simulink model "Ball_and_Plate_MicroLabBox_student"  (R2019b)
settings: Solver=ode1  StartTime=0.0  StopTime=Inf  FixedStep=0.001  RelTol=1e-3
PostLoadFcn:
  | , if any(exist('dsrtsu_mdlpostloadfcn', 'file') ~= 0), dsrtsu_mdlpostloadfcn('Execute', bdroot); end,
InitFcn:
  | , if any(exist('rtifpga_mdlclblib', 'file') ~= 0), rtifpga_mdlclblib('Init', bdroot); end,
undefined symbols (not defined in the file): A_obs, A_robust, B_obs, B_robust, ball_pos_sat, ball_vel_sat, C_obs, C_robust, D_obs, D_robust, g, K_lqr, path, plate_angle_sat, Q_kf, R_kf, Ts_fast, Ts_Inner, Ts_Outer, uA, uB, uC
libraries: rtiemclib x6, simulink x3, rtiethernetlib x3, rti1202lib_dac_class1 x3, mpclib x1
(part 3 of 3)

== matlab function Ball_and_Plate_MicroLabBox_student/Innerloop_Actuator/Motor_A/MATLAB Function ==
  data: e input; u output; reset_integrator input
function u = fcn(e, reset_integrator)
% You need to fill here

u = 0;

== matlab function Ball_and_Plate_MicroLabBox_student/Innerloop_Actuator/Motor_C/MATLAB Function ==
  data: e input; u output; reset_integrator input
function u = fcn(e, reset_integrator)
% You need to fill here

u = 0;

== matlab function Ball_and_Plate_MicroLabBox_student/Innerloop_Actuator/Motor_B/MATLAB Function1 ==
  data: e input; u output; reset_integrator input
function u = fcn(e, reset_integrator)
% You need to fill here

u = 0;

== matlab function Ball_and_Plate_MicroLabBox_student/Innerloop_Actuator/Motor_A/Multisine/MATLAB Function ==
  data: enable input; u input; y output
function y = Multisine_id(enable, u)

persistent index previous_enable

% Initialize
if isempty(index)
    index = 1;
end

if isempty(previous_enable)
    previous_enable = 0;
end

N = length(u);

% Detect rising edge (re-enable)
if enable && ~previous_enable
    index = 1;
end

% Output logic
if enable

    % If still inside signal → output sample
    if index <= N
        y = u(index);
        index = index + 1;

    else
        % Signal finished → output zero
        y = 0;
    end

else
    % Disabled → output zero
    y = 0;
end

previous_enable = enable;

== matlab function Ball_and_Plate_MicroLabBox_student/Innerloop_Actuator/Motor_B/Multisine/MATLAB Function ==
  data: enable input; u input; y output
function y = Multisine_id(enable, u)

persistent index previous_enable

% Initialize
if isempty(index)
    index = 1;
end

if isempty(previous_enable)
    previous_enable = 0;
end

N = length(u);

% Detect rising edge (re-enable)
if enable && ~previous_enable
    index = 1;
end

% Output logic
if enable

    % If still inside signal → output sample
    if index <= N
        y = u(index);
        index = index + 1;

    else
        % Signal finished → output zero
        y = 0;
    end

else
    % Disabled → output zero
    y = 0;
end

previous_enable = enable;

== matlab function Ball_and_Plate_MicroLabBox_student/Innerloop_Actuator/Motor_C/Multisine/MATLAB Function ==
  data: enable input; u input; y output
function y = Multisine_id(enable, u)

persistent index previous_enable

% Initialize
if isempty(index)
    index = 1;
end

if isempty(previous_enable)
    previous_enable = 0;
end

N = length(u);

% Detect rising edge (re-enable)
if enable && ~previous_enable
    index = 1;
end

% Output logic
if enable

    % If still inside signal → output sample
    if index <= N
        y = u(index);
        index = index + 1;

    else
        % Signal finished → output zero
        y = 0;
    end

else
    % Disabled → output zero
    y = 0;
end

previous_enable = enable;

== matlab function Ball_and_Plate_MicroLabBox_student/coordinates_ball ==
  data: x_2_pixels input; x_2 output; y_2_pixels input; y_2 output; theta_1 input; theta_2 input
function [x_2, y_2] = fcn(x_2_pixels, y_2_pixels, theta_1, theta_2)
    %A01_fun
    %    OUT1 = A01_fun(THETA_1,THETA_2)
    
    %    This function was generated by the Symbolic Math Toolbox version 9.3.
    %    22-May-2025 12:09:11
    y_offset = 242.82;
    x_offset = 295.83;
    conversion_factor = 1120.25;
%     ball_radius = 20e-3;%mm
    x_2_e0 = (double(x_2_pixels)-x_offset)/conversion_factor;
    y_2_e0 = (double(y_2_pixels)-y_offset)/conversion_factor;
    t2 = cos(theta_1);
    t3 = cos(theta_2);
    t4 = sin(theta_1);
    t5 = sin(theta_2);
    out1 = reshape([t3,t4.*t5,-t2.*t5,0.0,t2,t4,t5,-t3.*t4,t2.*t3],[3,3]);
%     temp = double([x_2_e0, y_2_e0, -ball_radius])*double(out1);
    x_2 = x_2_e0;%temp(1);
    y_2 = y_2_e0;%temp(2);
end

== matlab function Ball_and_Plate_MicroLabBox_student/Innerloop_Actuator/Motor_C/Multisine1/MATLAB Function ==
  data: enable input; u input; y output
function y = Multisine_id(enable, u)

persistent index previous_enable

% Initialize
if isempty(index)
    index = 1;
end

if isempty(previous_enable)
    previous_enable = 0;
end

N = length(u);

% Detect rising edge (re-enable)
if enable && ~previous_enable
    index = 1;
end

% Output logic
if enable

    % If still inside signal → output sample
    if index <= N
        y = u(index);
        index = index + 1;

    else
        % Signal finished → output zero
        y = 0;
    end

else
    % Disabled → output zero
    y = 0;
end

previous_enable = enable;

== matlab function Ball_and_Plate_MicroLabBox_student/Innerloop_Actuator/Motor_B/Init_motion/MATLAB Function1 ==
  data: reference_end input; path output; end_time input; Ts input; measured_position input
function path = Quintic_Polynomial_Trajectory_Time(reference_end, end_time, Ts, measured_position)
%% Quintic_Polynomial_Trajectory(reference_end, average_velocity)
% This function outputs a quintic polynomial trajectory over time in 
% Simulink given the end reference and average velocity. The starting 
% velocity and acceleration are set to zero.
%
% Input Arguments
% reference_end = desired end position of the trajectory
% end_time = end time of trajectory; for every new input 
% trajectory starts at time 0 and ends at end_time
% measured_position = current position of the robot arm
%
% Output Arguments
% path = path of the trajectory over time
%
% Quinten Swaan 17-08-2022
%
% Control Systems Technology group
% Departement of Mechanical Engineering
% Eindhoven University of Technology


persistent previous_value_reference_start previous_value_reference_end ...
    path_array index 

if isempty(previous_value_reference_start)
    previous_value_reference_start = 0;
end

if isempty(previous_value_reference_end)
    previous_value_reference_end = 0;
end

if isempty(path_array)
    path_array = zeros(1,1);
end

if isempty(index)
    index = 1;
end


% Obtain new trajectory if a new end reference is given
if previous_value_reference_end ~= reference_end
    t0 = 0;                                 %Starting time
    q0 = previous_value_reference_start;    %Starting position
    v0 = 0;                                 %Starting velocity
    ac0 = 0;                                %Starting acceleration
    tf = end_time;                          %End time
    qf = reference_end;                     %End position
    vf = 0;                                 %End velocity
    acf = 0;                                %End acceleration

    M = [1 t0 t0^2 t0^3 t0^4 t0^5;
    0 1 2*t0 3*t0^2 4*t0^3 5*t0^4;
    0 0 2 6*t0 12*t0^2 20*t0^3;
    1 tf tf^2 tf^3 tf^4 tf^5;
    0 1 2*tf 3*tf^2 4*tf^3 5*tf^4;
    0 0 2 6*tf 12*tf^2 20*tf^3];

    b = [q0; v0; ac0; qf; vf; acf];

    x = M \ b;

    t = t0:Ts:tf;

    path_array = x(1) + x(2).*t + x(3).*t.^2 + x(4).*t.^3 + +x(5).*t.^4 + x(6).*t.^5;

    index = 1;
    reference_current = path_array(index);

% Output the reference per timestep
else
    if index < length(path_array)
        index = index + 1;
    end
    reference_current = path_array(index);
end

previous_value_reference_end = reference_end;
previous_value_reference_start = measured_position;

path = reference_current;

== matlab function Ball_and_Plate_MicroLabBox_student/Innerloop_Actuator/Motor_B/Init_motion/MATLAB Function2 ==
  data: y input; path output; start input; init_value input; current_pos input
function path = init_motion(y, start, init_value, current_pos)

if start > 0.5
    path = init_value;
elseif start < 0.5
    path = y;
else 
    path = 0;
end

== matlab function Ball_and_Plate_MicroLabBox_student/Innerloop_Actuator/Motor_C/Init_motion/MATLAB Function1 ==
  data: reference_end input; path output; end_time input; Ts input; measured_position input
function path = Quintic_Polynomial_Trajectory_Time(reference_end, end_time, Ts, measured_position)
%% Quintic_Polynomial_Trajectory(reference_end, average_velocity)
% This function outputs a quintic polynomial trajectory over time in 
% Simulink given the end reference and average velocity. The starting 
% velocity and acceleration are set to zero.
%
% Input Arguments
% reference_end = desired end position of the trajectory
% end_time = end time of trajectory; for every new input 
% trajectory starts at time 0 and ends at end_time
% measured_position = current position of the robot arm
%
% Output Arguments
% path = path of the trajectory over time
%
% Quinten Swaan 17-08-2022
%
% Control Systems Technology group
% Departement of Mechanical Engineering
% Eindhoven University of Technology


persistent previous_value_reference_start previous_value_reference_end ...
    path_array index 

if isempty(previous_value_reference_start)
    previous_value_reference_start = 0;
end

if isempty(previous_value_reference_end)
    previous_value_reference_end = 0;
end

if isempty(path_array)
    path_array = zeros(1,1);
end

if isempty(index)
    index = 1;
end


% Obtain new trajectory if a new end reference is given
if previous_value_reference_end ~= reference_end
    t0 = 0;                                 %Starting time
    q0 = previous_value_reference_start;    %Starting position
    v0 = 0;                                 %Starting velocity
    ac0 = 0;                                %Starting acceleration
    tf = end_time;                          %End time
    qf = reference_end;                     %End position
    vf = 0;                                 %End velocity
    acf = 0;                                %End acceleration

    M = [1 t0 t0^2 t0^3 t0^4 t0^5;
    0 1 2*t0 3*t0^2 4*t0^3 5*t0^4;
    0 0 2 6*t0 12*t0^2 20*t0^3;
    1 tf tf^2 tf^3 tf^4 tf^5;
    0 1 2*tf 3*tf^2 4*tf^3 5*tf^4;
    0 0 2 6*tf 12*tf^2 20*tf^3];

    b = [q0; v0; ac0; qf; vf; acf];

    x = M \ b;

    t = t0:Ts:tf;

    path_array = x(1) + x(2).*t + x(3).*t.^2 + x(4).*t.^3 + +x(5).*t.^4 + x(6).*t.^5;

    index = 1;
    reference_current = path_array(index);

% Output the reference per timestep
else
    if index < length(path_array)
        index = index + 1;
    end
    reference_current = path_array(index);
end

previous_value_reference_end = reference_end;
previous_value_reference_start = measured_position;

path = reference_current;

== matlab function Ball_and_Plate_MicroLabBox_student/Innerloop_Actuator/Motor_C/Init_motion/MATLAB Function2 ==
  data: y input; path output; start input; init_value input; current_pos input
function path = init_motion(y, start, init_value, current_pos)

if start > 0.5
    path = init_value;
elseif start < 0.5
    path = y;
else 
    path = 0;
end

== matlab function Ball_and_Plate_MicroLabBox_student/Innerloop_Actuator/Motor_A/Init_motion/MATLAB Function ==
  data: enable input; u input; y output
function y = init_motion(enable, u)

persistent index previous_enable

% Initialize
if isempty(index)
    index = 1;
end

if isempty(previous_enable)
    previous_enable = 0;
end

N = length(u);

% Detect rising edge (re-enable)
if enable && ~previous_enable
    index = 1;
end

% Output logic
if enable

    % If still inside signal → output sample
    if index <= N
        y = u(index);
        index = index + 1;

    else
        % Signal finished → output zero
        y = 0;
    end

else
    % Disabled → output zero
    y = -0.0289;
end

previous_enable = enable;

== matlab function Ball_and_Plate_MicroLabBox_student/Innerloop_Actuator/Motor_B/Init_motion/MATLAB Function ==
  data: enable input; u input; y output
function y = init_motion(enable, u)

persistent index previous_enable

% Initialize
if isempty(index)
    index = 1;
end

if isempty(previous_enable)
    previous_enable = 0;
end

N = length(u);

% Detect rising edge (re-enable)
if enable && ~previous_enable
    index = 1;
end

% Output logic
if enable

    % If still inside signal → output sample
    if index <= N
        y = u(index);
        index = index + 1;

    else
        % Signal finished → output zero
        y = 0;
    end

else
    % Disabled → output zero
    y = -0.0289;
end

previous_enable = enable;

== matlab function Ball_and_Plate_MicroLabBox_student/Innerloop_Actuator/Motor_C/Init_motion/MATLAB Function ==
  data: enable input; u input; y output
function y = init_motion(enable, u)

persistent index previous_enable

% Initialize
if isempty(index)
    index = 1;
end

if isempty(previous_enable)
    previous_enable = 0;
end

N = length(u);

% Detect rising edge (re-enable)
if enable && ~previous_enable
    index = 1;
end

% Output logic
if enable

    % If still inside signal → output sample
    if index <= N
        y = u(index);
        index = index + 1;

    else
        % Signal finished → output zero
        y = 0;
    end

else
    % Disabled → output zero
    y = -0.0289;
end

previous_enable = enable;

== matlab function Ball_and_Plate_MicroLabBox_student/Innerloop_Actuator/AngleToPos  ==
  data: alpha input; pos1 output; beta input; psi input; pos2 output; pos3 output
function [pos1, pos2, pos3] = angleToPos(alpha, beta, psi)
    % Returns the actuator positions required to reach the desired angle
    % note: the position is absolute in the global frame

    % Physical Constants
    r = 0.17;           % Joint radius (m)
    T = [0; 0; 0.322];  % Resting height vector (m)
    
    % Joint positions on base and plate (equilateral triangle)
    % These match the definitions in your posToAngle function
    theta = [0, deg2rad(240), deg2rad(120)];
    B = [r*cos(theta); r*sin(theta); zeros(1,3)]; % Base joints (b_i)
    P = [r*cos(theta); r*sin(theta); zeros(1,3)]; % Plate joints (p_i)
    
    % Rotation Matrices (Yaw-Pitch-Roll order)
    Rz = [cos(psi) -sin(psi) 0; sin(psi) cos(psi) 0; 0 0 1];
    Ry = [cos(beta) 0 sin(beta); 0 1 0; -sin(beta) 0 cos(beta)];
    Rx = [1 0 0; 0 cos(alpha) -sin(alpha); 0 sin(alpha) cos(alpha)];
    R_BtoP = Rz * Ry * Rx; 
    
    % Compute absolute position for each motor
    % Motor 1
    l1_vec = T + (R_BtoP * P(:,1)) - B(:,1);
    pos1 = norm(l1_vec);
    
    % Motor 2
    l2_vec = T + (R_BtoP * P(:,2)) - B(:,2);
    pos2 = norm(l2_vec);
    
    % Motor 3
    l3_vec = T + (R_BtoP * P(:,3)) - B(:,3);
    pos3 = norm(l3_vec);
end

== matlab function Ball_and_Plate_MicroLabBox_student/Innerloop_Actuator/Motor_A/MATLAB Function1 ==
  data: reference_end input; path output; end_time input; Ts input; measured_position input
function path = Quintic_Time(reference_end, end_time, Ts, measured_position)
% QUINTIC_POLYNOMIAL_TRAJECTORY_TIME
% Calculated analytically per step to be compatible with dSPACE/Control Desk.

% Persistent variables to store coefficients and the "internal clock"
persistent coeffs t_elapsed prev_ref_end tf_internal
if isempty(coeffs)
    coeffs = zeros(6, 1); % a0, a1, a2, a3, a4, a5
end
if isempty(t_elapsed)
    t_elapsed = 0;
end
if isempty(prev_ref_end)
    prev_ref_end = reference_end;
end
if isempty(tf_internal)
    tf_internal = 0;
end

% Check if a new trajectory is requested
if reference_end ~= prev_ref_end
    % Reset timer
    t_elapsed = 0;
    tf_internal = end_time;
    
    % Boundary conditions
    q0 = prev_ref_end; 
    qf = reference_end;
    v0 = 0; vf = 0;
    ac0 = 0; acf = 0;
    
    % Solver for t0 = 0
    % We solve the system: M * coeffs = b
    % Using tf_internal instead of end_time to ensure consistency during the run
    T = tf_internal;
    M = [1, 0, 0,  0,    0,    0;
         0, 1, 0,  0,    0,    0;
         0, 0, 2,  0,    0,    0;
         1, T, T^2, T^3,  T^4,  T^5;
         0, 1, 2*T, 3*T^2, 4*T^3, 5*T^4;
         0, 0, 2,   6*T,   12*T^2, 20*T^3];
     
    b = [q0; v0; ac0; qf; vf; acf];
    
    % Calculate coefficients (Matrix is small 6x6, so this is fast)
    coeffs = M \ b;
end

% Calculate current reference based on elapsed time
t = t_elapsed;

if t <= tf_internal
    % Quintic Equation: path = a0 + a1*t + a2*t^2 + a3*t^3 + a4*t^4 + a5*t^5
    path = coeffs(1) + coeffs(2)*t + coeffs(3)*t^2 + coeffs(4)*t^3 + coeffs(5)*t^4 + coeffs(6)*t^5;
    
    % Increment time for the next step
    t_elapsed = t_elapsed + Ts;
else
    % Hold the final position once trajectory is finished
    path = reference_end;
end

% Update memory for next iteration
prev_ref_end = reference_end;

end

== matlab function Ball_and_Plate_MicroLabBox_student/Innerloop_Actuator/Motor_B/MATLAB Function2 ==
  data: reference_end input; path output; end_time input; Ts input; measured_position input
function path = Quintic_Time(reference_end, end_time, Ts, measured_position)
% QUINTIC_POLYNOMIAL_TRAJECTORY_TIME
% Calculated analytically per step to be compatible with dSPACE/Control Desk.

% Persistent variables to store coefficients and the "internal clock"
persistent coeffs t_elapsed prev_ref_end tf_internal
if isempty(coeffs)
    coeffs = zeros(6, 1); % a0, a1, a2, a3, a4, a5
end
if isempty(t_elapsed)
    t_elapsed = 0;
end
if isempty(prev_ref_end)
    prev_ref_end = reference_end;
end
if isempty(tf_internal)
    tf_internal = 0;
end

% Check if a new trajectory is requested
if reference_end ~= prev_ref_end
    % Reset timer
    t_elapsed = 0;
    tf_internal = end_time;
    
    % Boundary conditions
    q0 = prev_ref_end; 
    qf = reference_end;
    v0 = 0; vf = 0;
    ac0 = 0; acf = 0;
    
    % Solver for t0 = 0
    % We solve the system: M * coeffs = b
    % Using tf_internal instead of end_time to ensure consistency during the run
    T = tf_internal;
    M = [1, 0, 0,  0,    0,    0;
         0, 1, 0,  0,    0,    0;
         0, 0, 2,  0,    0,    0;
         1, T, T^2, T^3,  T^4,  T^5;
         0, 1, 2*T, 3*T^2, 4*T^3, 5*T^4;
         0, 0, 2,   6*T,   12*T^2, 20*T^3];
     
    b = [q0; v0; ac0; qf; vf; acf];
    
    % Calculate coefficients (Matrix is small 6x6, so this is fast)
    coeffs = M \ b;
end

% Calculate current reference based on elapsed time
t = t_elapsed;

if t <= tf_internal
    % Quintic Equation: path = a0 + a1*t + a2*t^2 + a3*t^3 + a4*t^4 + a5*t^5
    path = coeffs(1) + coeffs(2)*t + coeffs(3)*t^2 + coeffs(4)*t^3 + coeffs(5)*t^4 + coeffs(6)*t^5;
    
    % Increment time for the next step
    t_elapsed = t_elapsed + Ts;
else
    % Hold the final position once trajectory is finished
    path = reference_end;
end

% Update memory for next iteration
prev_ref_end = reference_end;

end

== matlab function Ball_and_Plate_MicroLabBox_student/Innerloop_Actuator/Motor_C/MATLAB Function1 ==
  data: reference_end input; path output; end_time input; Ts input; measured_position input
function path = Quintic_Time(reference_end, end_time, Ts, measured_position)
% QUINTIC_POLYNOMIAL_TRAJECTORY_TIME
% Calculated analytically per step to be compatible with dSPACE/Control Desk.

% Persistent variables to store coefficients and the "internal clock"
persistent coeffs t_elapsed prev_ref_end tf_internal
if isempty(coeffs)
    coeffs = zeros(6, 1); % a0, a1, a2, a3, a4, a5
end
if isempty(t_elapsed)
    t_elapsed = 0;
end
if isempty(prev_ref_end)
    prev_ref_end = reference_end;
end
if isempty(tf_internal)
    tf_internal = 0;
end

% Check if a new trajectory is requested
if reference_end ~= prev_ref_end
    % Reset timer
    t_elapsed = 0;
    tf_internal = end_time;
    
    % Boundary conditions
    q0 = prev_ref_end; 
    qf = reference_end;
    v0 = 0; vf = 0;
    ac0 = 0; acf = 0;
    
    % Solver for t0 = 0
    % We solve the system: M * coeffs = b
    % Using tf_internal instead of end_time to ensure consistency during the run
    T = tf_internal;
    M = [1, 0, 0,  0,    0,    0;
         0, 1, 0,  0,    0,    0;
         0, 0, 2,  0,    0,    0;
         1, T, T^2, T^3,  T^4,  T^5;
         0, 1, 2*T, 3*T^2, 4*T^3, 5*T^4;
         0, 0, 2,   6*T,   12*T^2, 20*T^3];
     
    b = [q0; v0; ac0; qf; vf; acf];
    
    % Calculate coefficients (Matrix is small 6x6, so this is fast)
    coeffs = M \ b;
end

% Calculate current reference based on elapsed time
t = t_elapsed;

if t <= tf_internal
    % Quintic Equation: path = a0 + a1*t + a2*t^2 + a3*t^3 + a4*t^4 + a5*t^5
    path = coeffs(1) + coeffs(2)*t + coeffs(3)*t^2 + coeffs(4)*t^3 + coeffs(5)*t^4 + coeffs(6)*t^5;
    
    % Increment time for the next step
    t_elapsed = t_elapsed + Ts;
else
    % Hold the final position once trajectory is finished
    path = reference_end;
end

% Update memory for next iteration
prev_ref_end = reference_end;

end

== matlab function Ball_and_Plate_MicroLabBox_student/Ethernet communication/MATLAB Function ==
  data: x output; u input; y output; z output; flag output
function [x,y,z,flag] = fcn(u)
    x = double(u(1)) + 256*double(u(2));
    y = double(u(5)) + 256*double(u(6));
    z = double(u(9)) + 256*double(u(10));
    flag = u(11);
    
    if x > 32767
        x = x-65536;
    end
    if y > 32767
        y = y-65536;
    end
    if z > 32767
        z = z-65536;
    end
end

== matlab function Ball_and_Plate_MicroLabBox_student/Innerloop_Actuator/PosToAngle  ==
  data: pos1 input; alpha output; pos2 input; pos3 input; beta output; psi output
function [alpha, beta, psi] = posToAngle(pos1, pos2, pos3)
    % Returns the angles resulting from the given position
    % note: the position should be relative from the actuators midpoint in the global frame

    % Physical Constants
    r = 0.17;                 % Radius to joints (m)
    T = 0.322;                % Resting height (m)
    theta = deg2rad(120);     % angle between bases (rad)

    % Reconstruction of the Plate Unit Vectors 
    % We find where the joints are in the world frame by using the inputs
    % If pos = 0.322, the joints are exactly T_height above the base.
    P1_global = [r; 0; T + pos1];
    P2_global = [r*cos(theta); r*sin(theta); T + pos2];
    P3_global = [r*cos(theta); -r*sin(theta); T + pos3];

    % Find the center of the tilted plate
    % The average of the three joint positions gives the center of the motion plate
    center = (P1_global + P2_global + P3_global) / 3;

    % Vectors from the plate center to the joints
    % This isolates the tilt of the plate surface
    v1 = P1_global - center;
    v2 = P2_global - center;
    v3 = P3_global - center;

    % Compute Unit Vectors
    uX = v1 / norm(v1);             % Plate X-axis
    u_temp = cross(uX, v3);         % Temporary vector to find normal
    uZ = u_temp / norm(u_temp);     % Plate Z-axis (Normal)
    uY = cross(uZ, uX);             % Plate Y-axis

    % Extract Tait-Bryan Angles
    beta = asin(-uX(3));                            
    alpha = asin(uY(3) / sqrt(1 - uX(3)^2));       
    psi = asin(uX(2) / sqrt(1 - uX(3)^2));
end

== matlab function Ball_and_Plate_MicroLabBox_student/MATLAB Function ==
  data: y_meas input; u input; x_est output; valid_frame input; Qkf input; Rkf input; Ts input
function x_est = intermittent_kalman(y_meas, u, valid_frame, Qkf, Rkf, Ts)
    
    g = 9.81;
    Ad = [1, Ts, 0,0;
        0, 1, 0, 0;
        0, 0, 1, Ts;
        0, 0, 0, 1];

    Bd = [5/14 * g * Ts^2, 0;
        5/7 * g * Ts, 0;
        0, 5/14 * g * Ts^2;
        0, 5/7 * g * Ts];
    
    Cd = [1 0 0 0;
        0 0 1 0];


    % Persistent variables keep their state between sample steps
    persistent x_hat P
    
    % Initialization on the very first time step
    if isempty(x_hat)
        x_hat = zeros(4,1);
        P = eye(4) * 0.1;
    end
    
    % 1. Prediction Step (Always executes)
    x_pred = Ad * x_hat + Bd * u;
    P_pred = Ad * P * Ad' + Qkf;
    
    % 2. Correction Step (Conditional)
    if valid_frame > 0.5
        % Frame is valid: Run normal Kalman Correction
        S = Cd * P_pred * Cd' + Rkf;
        K = P_pred * Cd' / S; % Equivalent to P_pred * Cd' * inv(S)
        
        x_hat = x_pred + K * (y_meas - Cd * x_pred);
        P = (eye(4) - K * Cd) * P_pred;
    else
        % Frame was dropped: Skip correction, trust physics prediction
        x_hat = x_pred;
        P = P_pred;
    end
    
    % Output the current state estimate
    x_est = x_hat;
end

== matlab function Ball_and_Plate_MicroLabBox_student/MATLAB Function1 ==
  data: reference_end input; path output; end_time input; Ts input; measured_position input
function path = Quintic_Time(reference_end, end_time, Ts, measured_position)
% QUINTIC_POLYNOMIAL_TRAJECTORY_TIME
% Calculated analytically per step to be compatible with dSPACE/Control Desk.

% Persistent variables to store coefficients and the "internal clock"
persistent coeffs t_elapsed prev_ref_end tf_internal
if isempty(coeffs)
    coeffs = zeros(6, 1); % a0, a1, a2, a3, a4, a5
end
if isempty(t_elapsed)
    t_elapsed = 0;
end
if isempty(prev_ref_end)
    prev_ref_end = reference_end;
end
if isempty(tf_internal)
    tf_internal = 0;
end

% Check if a new trajectory is requested
if reference_end ~= prev_ref_end
    % Reset timer
    t_elapsed = 0;
    tf_internal = end_time;
    
    % Boundary conditions
    q0 = prev_ref_end; 
    qf = reference_end;
    v0 = 0; vf = 0;
    ac0 = 0; acf = 0;
    
    % Solver for t0 = 0
    % We solve the system: M * coeffs = b
    % Using tf_internal instead of end_time to ensure consistency during the run
    T = tf_internal;
    M = [1, 0, 0,  0,    0,    0;
         0, 1, 0,  0,    0,    0;
         0, 0, 2,  0,    0,    0;
         1, T, T^2, T^3,  T^4,  T^5;
         0, 1, 2*T, 3*T^2, 4*T^3, 5*T^4;
         0, 0, 2,   6*T,   12*T^2, 20*T^3];
     
    b = [q0; v0; ac0; qf; vf; acf];
    
    % Calculate coefficients (Matrix is small 6x6, so this is fast)
    coeffs = M \ b;
end

% Calculate current reference based on elapsed time
t = t_elapsed;

if t <= tf_internal
    % Quintic Equation: path = a0 + a1*t + a2*t^2 + a3*t^3 + a4*t^4 + a5*t^5
    path = coeffs(1) + coeffs(2)*t + coeffs(3)*t^2 + coeffs(4)*t^3 + coeffs(5)*t^4 + coeffs(6)*t^5;
    
    % Increment time for the next step
    t_elapsed = t_elapsed + Ts;
else
    % Hold the final position once trajectory is finished
    path = reference_end;
end

% Update memory for next iteration
prev_ref_end = reference_end;

end

== matlab function Ball_and_Plate_MicroLabBox_student/MATLAB Function2 ==
  data: reference_end input; path output; end_time input; Ts input; measured_position input
function path = Quintic_Time(reference_end, end_time, Ts, measured_position)
% QUINTIC_POLYNOMIAL_TRAJECTORY_TIME
% Calculated analytically per step to be compatible with dSPACE/Control Desk.

% Persistent variables to store coefficients and the "internal clock"
persistent coeffs t_elapsed prev_ref_end tf_internal
if isempty(coeffs)
    coeffs = zeros(6, 1); % a0, a1, a2, a3, a4, a5
end
if isempty(t_elapsed)
    t_elapsed = 0;
end
if isempty(prev_ref_end)
    prev_ref_end = reference_end;
end
if isempty(tf_internal)
    tf_internal = 0;
end

% Check if a new trajectory is requested
if reference_end ~= prev_ref_end
    % Reset timer
    t_elapsed = 0;
    tf_internal = end_time;
    
    % Boundary conditions
    q0 = prev_ref_end; 
    qf = reference_end;
    v0 = 0; vf = 0;
    ac0 = 0; acf = 0;
    
    % Solver for t0 = 0
    % We solve the system: M * coeffs = b
    % Using tf_internal instead of end_time to ensure consistency during the run
    T = tf_internal;
    M = [1, 0, 0,  0,    0,    0;
         0, 1, 0,  0,    0,    0;
         0, 0, 2,  0,    0,    0;
         1, T, T^2, T^3,  T^4,  T^5;
         0, 1, 2*T, 3*T^2, 4*T^3, 5*T^4;
         0, 0, 2,   6*T,   12*T^2, 20*T^3];
     
    b = [q0; v0; ac0; qf; vf; acf];
    
    % Calculate coefficients (Matrix is small 6x6, so this is fast)
    coeffs = M \ b;
end

% Calculate current reference based on elapsed time
t = t_elapsed;

if t <= tf_internal
    % Quintic Equation: path = a0 + a1*t + a2*t^2 + a3*t^3 + a4*t^4 + a5*t^5
    path = coeffs(1) + coeffs(2)*t + coeffs(3)*t^2 + coeffs(4)*t^3 + coeffs(5)*t^4 + coeffs(6)*t^5;
    
    % Increment time for the next step
    t_elapsed = t_elapsed + Ts;
else
    % Hold the final position once trajectory is finished
    path = reference_end;
end

% Update memory for next iteration
prev_ref_end = reference_end;

end

== matlab function Ball_and_Plate_MicroLabBox_student/MATLAB Function3 ==
  data: R input; r output; omega input; Ts input; enable input
function r = Circle_Reference_spiral(R, omega, Ts, enable)
% CIRCLE_REFERENCE Generates [x; xdot; y; ydot] for a spiral-in/spiral-out trajectory.

% Persistent variables to track phase and the dynamic radius
persistent theta current_R

% Initialize persistent variables on the very first run
if isempty(theta)
    theta = 0;
end
if isempty(current_R)
    current_R = 0; % Start at the origin (0,0)
end

% Define how long you want the spiral transition to take (in seconds)
T_ramp = 5.0; 
R_rate = R / T_ramp; % Radial speed (units per second)

% Determine target radius based on the reset flag
if enable
    R_target = R;  % Spiral inward to origin
else
    R_target = 0;  % Spiral outward to full circle
end

% Smoothly update the current radius and compute dR (radial velocity)
if current_R < R_target
    dR = R_rate;
    current_R = current_R + dR * Ts;
    if current_R > R_target
        current_R = R_target;
        dR = 0;
    end
elseif current_R > R_target
    dR = -R_rate;
    current_R = current_R + dR * Ts;
    if current_R < R_target
        current_R = R_target;
        dR = 0;
    end
else
    dR = 0; % Radius is at target, no radial velocity
end

% Compute current positions and velocities
% Note: Velocities now include the dR component for perfect kinematic accuracy!
x     = current_R * cos(theta);
x_dot = dR * cos(theta) - current_R * omega * sin(theta);

y     = current_R * sin(theta);
y_dot = dR * sin(theta) + current_R * omega * cos(theta);

r = [x; x_dot; y; y_dot];

% Integrate the phase for the next time step
next_theta = theta + omega * Ts;

% Wrap theta to [0, 2*pi] to protect numerical precision
theta = mod(next_theta, 2*pi);
end
